simulink model "SimpleMessagesPortValueModel"  (R2020a)
settings: Solver=VariableStepAuto  StartTime=0.0  StopTime=10.0  RelTol=1e-3
InitFcn:
  | load('Data_message.mat');
libraries: simulink x1
settings Model: Creator=The MathWorks, Inc.  LastModifiedBy=The MathWorks, Inc.

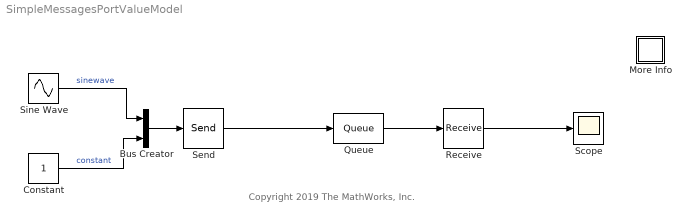
== system SimpleMessagesPortValueModel ==
  note: Copyright 2019 The MathWorks, Inc.
  Bus Creator : BusCreator  Inputs=2  OutDataTypeStr=Bus: Data_message  NonVirtualBus=on
      settings: InheritFromInputs=off
  Constant : Constant
  More Info : Subsystem
      settings: OpenFcn=showExample('simulink/ModelMessageBasedCommunicationFrameworkExample')
      mask Display: disp('?')
  Queue : Queue  InputPortMessageModes=m  OutputPortMessageModes=m  OverwriteOldest=on  Capacity=16  QueueType=LIFO
  Receive : Receive  InputPortMessageModes=m  UseInternalQueue=off  QueueOverwriting=on  QueueLength=1  QueueType=LIFO  SampleTime=0.1
  Scope : Scope
  Send : Send  OutputPortMessageModes=m
  Sine Wave : Sin  SampleTime=0.1
  wires:
  Receive/1 -> Scope/1
  Queue/1 -> Receive/1
  Send/1 -> Queue/1
  Sine Wave/1 -> Bus Creator/1  "sinewave"
  Bus Creator/1 -> Send/1
  Constant/1 -> Bus Creator/2  "constant"

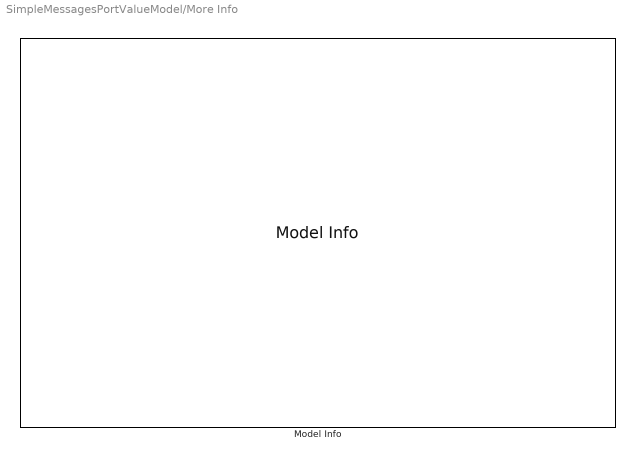
== system SimpleMessagesPortValueModel/More Info ==
  Model Info : simulink/Model-Wide Utilities/Model Info  Frame=on  DisplayStringWithTags=|  HorizontalTextAlignment=Left  LeftAlignmentValue=0.02
      | Model Description:
      | -------------------
      | This example shows how to use the Message Delay block to model a variable
      | speed conveyor belt between two airport terminals. The passengers step on
      | the conveyor belt following a Poisson distribution. Since passengers are
      | discrete entities, they are naturally modeled by Simulink(R) messages,
      | which are created by the Entity Generator block. When a passenger, i.e.,
      | a Simulink(R) message, is sent to the Message Delay block, the block
      | will hold it until it arrives at the other end of the conveyor belt. The
      | length of the delay time is automatically calculated by Simulink(R) based
      | on the ETA (estimated time of arrival), which is calculated by the
      | Stateflow(R) Chart. The operation of the conveyor belt depends on the
      | load and its transfer characteristics.
